simulink model "three_phase_PMSM"  (R2017b)
settings: Solver=VariableStepAuto  StartTime=0.0  StopTime=100  RelTol=1e-3
values from neighbouring files (symbols this model uses):
  J = 1    [three_phase_PMSM_parameters.m]
  M = 0    [three_phase_PMSM_parameters.m]
  psi_f = 1    [three_phase_PMSM_parameters.m]
  Rs = 10    [three_phase_PMSM_parameters.m]
  Z = 1    [three_phase_PMSM_parameters.m]
undefined symbols (not defined in the file or in its folder): Lsd, Lsq
settings Model: Creator=Алексей  LastModifiedBy=Алексей

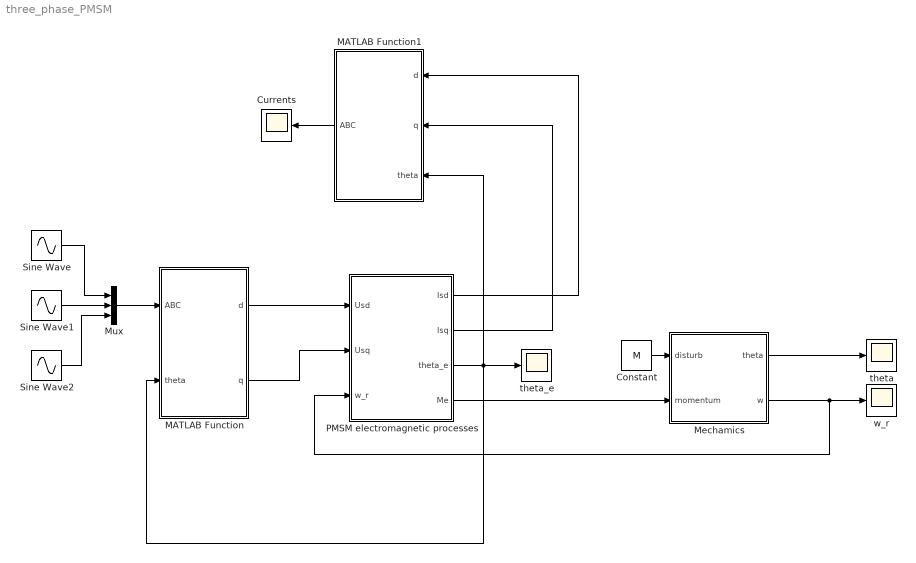
== system three_phase_PMSM ==
  Constant : Constant  Value=M
  Currents : Scope
  MATLAB Function : MATLAB Function  TreatAsAtomicUnit=on
  MATLAB Function1 : MATLAB Function  TreatAsAtomicUnit=on
  Mechamics : Subsystem
  Mux : Mux  Inputs=3
  PMSM electromagnetic processes : Subsystem
  Sine Wave : Sin  Amplitude=50  Frequency=50  SampleTime=0
  Sine Wave1 : Sin  Amplitude=50  Frequency=50  Phase=2*pi/3  SampleTime=0
  Sine Wave2 : Sin  Amplitude=50  Frequency=50  Phase=-2*pi/3  SampleTime=0
  theta : Scope
  theta_e : Scope
  w_r : Scope
  wires:
  Constant/1 -> Mechamics/1(disturb)
  PMSM electromagnetic processes/4(Me) -> Mechamics/2(momentum)
  Mechamics/2(w) -> w_r/1, PMSM electromagnetic processes/3(w_r)
  Mechamics/1(theta) -> theta/1
  PMSM electromagnetic processes/3(theta_e) -> MATLAB Function1/3(theta), MATLAB Function/2(theta), theta_e/1
  Sine Wave/1 -> Mux/1
  Sine Wave1/1 -> Mux/2
  Sine Wave2/1 -> Mux/3
  Mux/1 -> MATLAB Function/1(ABC)
  MATLAB Function/1(d) -> PMSM electromagnetic processes/1(Usd)
  MATLAB Function/2(q) -> PMSM electromagnetic processes/2(Usq)
  PMSM electromagnetic processes/1(Isd) -> MATLAB Function1/1(d)
  PMSM electromagnetic processes/2(Isq) -> MATLAB Function1/2(q)
  MATLAB Function1/1(ABC) -> Currents/1

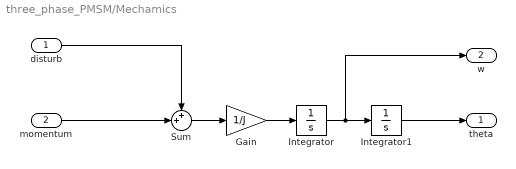
== system three_phase_PMSM/Mechamics ==
  disturb : Inport
  momentum : Inport  Port=2
  Gain : Gain  Gain=1/J
  Integrator : Integrator
  Integrator1 : Integrator
  Sum : Sum  Inputs=++|
  theta : Outport
  w : Outport  Port=2
  wires:
  Integrator/1 -> w/1, Integrator1/1
  disturb/1 -> Sum/1
  momentum/1 -> Sum/2
  Integrator1/1 -> theta/1
  Sum/1 -> Gain/1
  Gain/1 -> Integrator/1

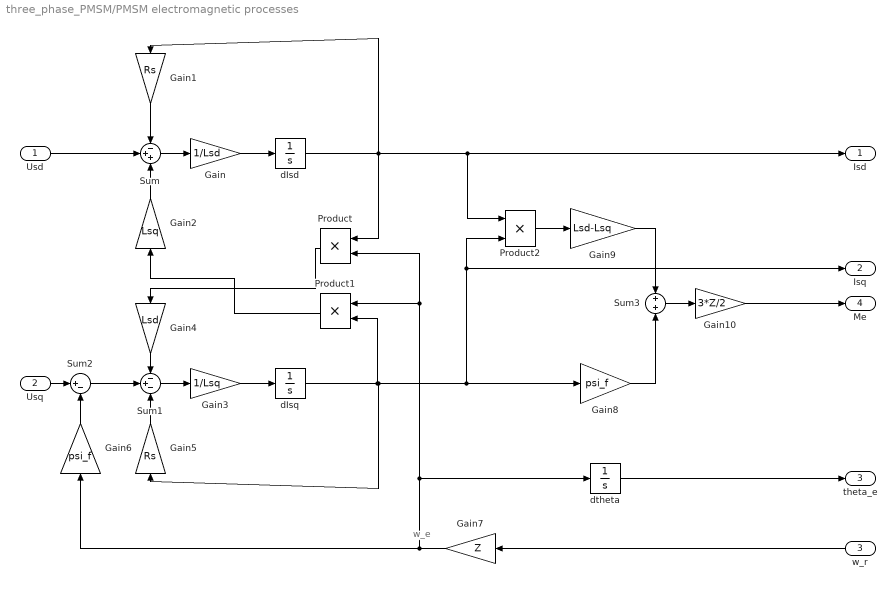
== system three_phase_PMSM/PMSM electromagnetic processes ==
  note: w_e
  Usd : Inport
  Usq : Inport  Port=2
  w_r : Inport  Port=3
  Gain : Gain  Gain=1/Lsd
  Gain1 : Gain  Gain=Rs
  Gain10 : Gain  Gain=3*Z/2
  Gain2 : Gain  Gain=Lsq
  Gain3 : Gain  Gain=1/Lsq
  Gain4 : Gain  Gain=Lsd
  Gain5 : Gain  Gain=Rs
  Gain6 : Gain  Gain=psi_f
  Gain7 : Gain  Gain=Z
  Gain8 : Gain  Gain=psi_f
  Gain9 : Gain  Gain=Lsd-Lsq
  Product : Product
  Product1 : Product
  Product2 : Product
  Sum : Sum  Inputs=-++
  Sum1 : Sum  Inputs=-+-
  Sum2 : Sum  Inputs=|+-
  Sum3 : Sum
  dIsd : Integrator
  dIsq : Integrator
  dtheta : Integrator
  Isd : Outport
  Isq : Outport  Port=2
  theta_e : Outport  Port=3
  Me : Outport  Port=4
  wires:
  dtheta/1 -> theta_e/1
  w_r/1 -> Gain7/1
  Usd/1 -> Sum/2
  Usq/1 -> Sum2/1
  Gain10/1 -> Me/1
  Gain8/1 -> Sum3/2
  Gain7/1 -> dtheta/1, Product1/1, Product/2, Gain6/1
  Product2/1 -> Gain9/1
  Product1/1 -> Gain2/1
  dIsd/1 -> Isd/1, Product2/1, Product/1, Gain1/1
  Gain/1 -> dIsd/1
  Gain1/1 -> Sum/1
  Sum3/1 -> Gain10/1
  Gain5/1 -> Sum1/3
  Sum/1 -> Gain/1
  Gain2/1 -> Sum/3
  dIsq/1 -> Product1/2, Gain8/1, Product2/2, Isq/1, Gain5/1
  Gain9/1 -> Sum3/1
  Gain6/1 -> Sum2/2
  Product/1 -> Gain4/1
  Gain3/1 -> dIsq/1
  Sum1/1 -> Gain3/1
  Sum2/1 -> Sum1/2
  Gain4/1 -> Sum1/1

== matlab function three_phase_PMSM/MATLAB Function1 ==
  data: d input; q input; ABC output; theta input
function ABC  = dq_ABC(d, q, theta)
A = d*cos(theta)-q*sin(theta);
B = sqrt(3)/2*(q*cos(theta)+d*sin(theta))-0.5*A;
C = -sqrt(3)/2*(q*cos(theta)+d*sin(theta))-0.5*A;

ABC=[A; B; C];

== matlab function three_phase_PMSM/MATLAB Function ==
  data: ABC input; d output; theta input; q output
function [d, q] = ABC_dq(ABC, theta)
A = ABC(1);
B = ABC(2);
C = ABC(3);

d = (B-C)/sqrt(3)*sin(theta)+A*cos(theta);
q = (B-C)/sqrt(3)*cos(theta)-A*sin(theta);
